simulink model "pm"  (R2023b)
settings: Solver=VariableStepAuto  StartTime=0.0  StopTime=10.0  MaxStep=0.001  RelTol=1e-3
settings Model: Creator=ASUS  LastModifiedBy=ASUS

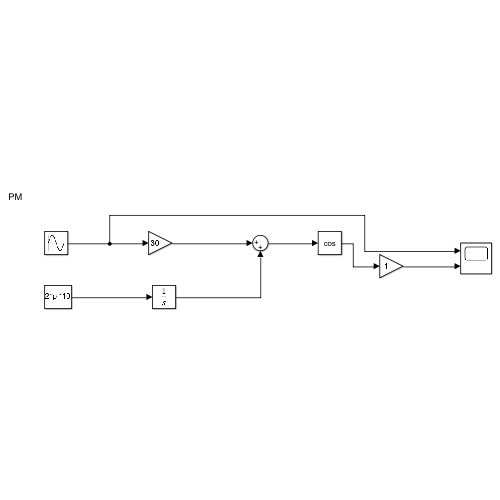
[thumbnail: Simulink's stored preview of the top-level diagram]
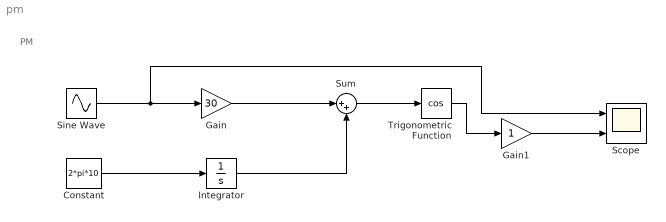
== system pm ==
  note: PM
  Constant : Constant  Value=2*pi*10
  Gain : Gain  Gain=30
  Gain1 : Gain
  Integrator : Integrator
  Scope : Scope  NumInputPorts=2
  Sine Wave : Sin  Frequency=1*2*pi  SampleTime=0
  Sum : Sum  Inputs=|++
  Trigonometric Function : Trigonometry  Operator=cos
  wires:
  Constant/1 -> Integrator/1
  Sine Wave/1 -> Scope/1, Gain/1
  Gain/1 -> Sum/1
  Integrator/1 -> Sum/2
  Sum/1 -> Trigonometric Function/1
  Trigonometric Function/1 -> Gain1/1
  Gain1/1 -> Scope/2
